simulink model "czujniki"  (R2013a)
settings: Solver=ode4  StartTime=0.0  StopTime=10  FixedStep=0.1  RelTol=1e-3
undefined symbols (not defined in the file or in its folder): serial
libraries: instrumentlib x2, dspindex x1
settings Model: Creator=Dzientak  LastModifiedBy=Dzientak

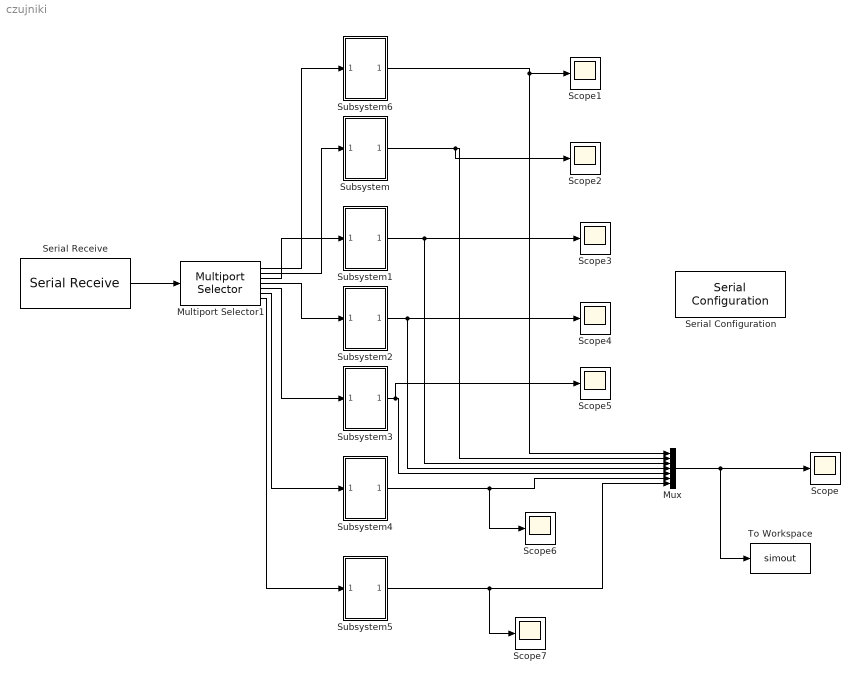
== system czujniki ==
  Multiport Selector1 : dspindex/Multiport Selector  rowsOrCols=Columns  idxCellArray={1,2,3,4,5,6,7 }  idxErrMode=Clip Index
  Mux : Mux  Inputs=7
  Scope{,1..7} (8 alike) : Scope
      Scope2 settings: SaveName=ScopeData2
      Scope3 settings: SaveName=ScopeData3
      Scope4 settings: SaveName=ScopeData4
      Scope5 settings: SaveName=ScopeData5
      Scope6 settings: SaveName=ScopeData6
      Scope7 settings: SaveName=ScopeData7
  Serial Configuration : instrumentlib/Serial Configuration  Priority=-200000  ComPortMenu=COM7  ComPort=COM7  ObjConstructor=serial('COM7');  BaudRate=9600  DataBits=8  Parity=none  StopBits=1  FlowControl=none  Timeout=10  ByteOrder=LittleEndian
  Serial Receive : instrumentlib/Serial Receive  ComPortMenu=COM7  ComPort=COM7  ObjConstructor=serial('COM7');  Terminator=<none>  DataSize="[8  7]"  DataType=uint8  EnableBlockingMode=on  ActionDataUnavailable=Output last received value  CustomValue=0  SampleTime=0.1
  Subsystem : Subsystem
  Subsystem1 : Subsystem
  Subsystem2 : Subsystem
  Subsystem3 : Subsystem
  Subsystem4 : Subsystem
  Subsystem5 : Subsystem
  Subsystem6 : Subsystem
  To Workspace : ToWorkspace  VariableName=simout  SampleTime=-1
  wires:
  Serial Receive/1 -> Multiport Selector1/1
  Multiport Selector1/1 -> Subsystem6/1(In1)
  Multiport Selector1/2 -> Subsystem/1(In1)
  Multiport Selector1/3 -> Subsystem1/1(In1)
  Multiport Selector1/4 -> Subsystem2/1(In1)
  Multiport Selector1/5 -> Subsystem3/1(In1)
  Multiport Selector1/6 -> Subsystem4/1(In1)
  Multiport Selector1/7 -> Subsystem5/1(In1)
  Subsystem6/1(Out1) -> Scope1/1, Mux/1
  Subsystem/1(Out1) -> Scope2/1, Mux/2
  Subsystem1/1(Out1) -> Scope3/1, Mux/3
  Subsystem2/1(Out1) -> Scope4/1, Mux/4
  Subsystem3/1(Out1) -> Scope5/1, Mux/5
  Subsystem4/1(Out1) -> Scope6/1, Mux/6
  Mux/1 -> To Workspace/1, Scope/1
  Subsystem5/1(Out1) -> Scope7/1, Mux/7

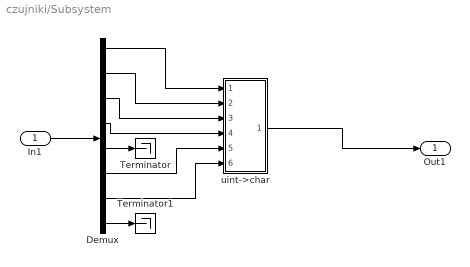
== system czujniki/Subsystem ==
  In1 : Inport
  Demux : Demux  Outputs=8
  Terminator : Terminator
  Terminator1 : Terminator
  uint->char : Subsystem
  Out1 : Outport
  wires:
  In1/1 -> Demux/1
  Demux/8 -> Terminator1/1
  Demux/5 -> Terminator/1
  Demux/7 -> uint->char/6(In6)
  Demux/6 -> uint->char/5(In5)
  Demux/4 -> uint->char/4(In4)
  Demux/3 -> uint->char/3(In3)
  Demux/2 -> uint->char/2(In2)
  Demux/1 -> uint->char/1(In1)
  uint->char/1(Out1) -> Out1/1

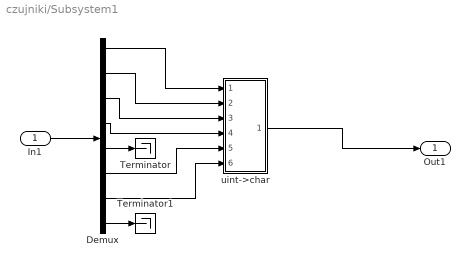
== system czujniki/Subsystem1 ==
  In1 : Inport
  Demux : Demux  Outputs=8
  Terminator : Terminator
  Terminator1 : Terminator
  uint->char : Subsystem
  Out1 : Outport
  wires:
  uint->char/1(Out1) -> Out1/1
  Demux/1 -> uint->char/1(In1)
  Demux/2 -> uint->char/2(In2)
  Demux/3 -> uint->char/3(In3)
  Demux/4 -> uint->char/4(In4)
  Demux/6 -> uint->char/5(In5)
  Demux/7 -> uint->char/6(In6)
  Demux/5 -> Terminator/1
  Demux/8 -> Terminator1/1
  In1/1 -> Demux/1

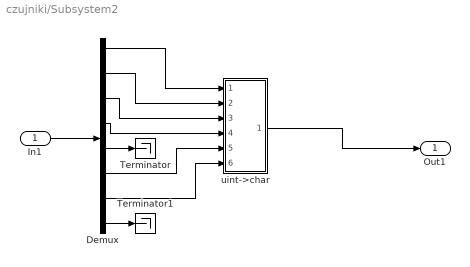
== system czujniki/Subsystem2 ==
  In1 : Inport
  Demux : Demux  Outputs=8
  Terminator : Terminator
  Terminator1 : Terminator
  uint->char : Subsystem
  Out1 : Outport
  wires:
  In1/1 -> Demux/1
  Demux/8 -> Terminator1/1
  Demux/5 -> Terminator/1
  Demux/7 -> uint->char/6(In6)
  Demux/6 -> uint->char/5(In5)
  Demux/4 -> uint->char/4(In4)
  Demux/3 -> uint->char/3(In3)
  Demux/2 -> uint->char/2(In2)
  Demux/1 -> uint->char/1(In1)
  uint->char/1(Out1) -> Out1/1

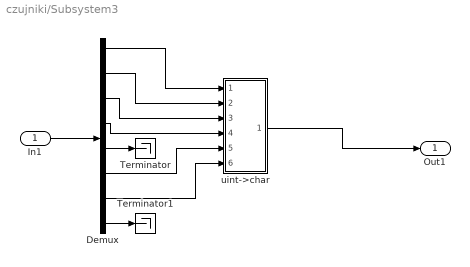
== system czujniki/Subsystem3 ==
  In1 : Inport
  Demux : Demux  Outputs=8
  Terminator : Terminator
  Terminator1 : Terminator
  uint->char : Subsystem
  Out1 : Outport
  wires:
  uint->char/1(Out1) -> Out1/1
  Demux/1 -> uint->char/1(In1)
  Demux/2 -> uint->char/2(In2)
  Demux/3 -> uint->char/3(In3)
  Demux/4 -> uint->char/4(In4)
  Demux/6 -> uint->char/5(In5)
  Demux/7 -> uint->char/6(In6)
  Demux/5 -> Terminator/1
  Demux/8 -> Terminator1/1
  In1/1 -> Demux/1

== system czujniki/Subsystem4 ==
  In1 : Inport
  Demux : Demux  Outputs=8
  Terminator : Terminator
  Terminator1 : Terminator
  uint->char : Subsystem
  Out1 : Outport
  wires:
  In1/1 -> Demux/1
  Demux/8 -> Terminator1/1
  Demux/5 -> Terminator/1
  Demux/7 -> uint->char/6(In6)
  Demux/6 -> uint->char/5(In5)
  Demux/4 -> uint->char/4(In4)
  Demux/3 -> uint->char/3(In3)
  Demux/2 -> uint->char/2(In2)
  Demux/1 -> uint->char/1(In1)
  uint->char/1(Out1) -> Out1/1

== system czujniki/Subsystem5 ==
  In1 : Inport
  Demux : Demux  Outputs=8
  Terminator : Terminator
  Terminator1 : Terminator
  uint->char : Subsystem
  Out1 : Outport
  wires:
  uint->char/1(Out1) -> Out1/1
  Demux/1 -> uint->char/1(In1)
  Demux/2 -> uint->char/2(In2)
  Demux/3 -> uint->char/3(In3)
  Demux/4 -> uint->char/4(In4)
  Demux/6 -> uint->char/5(In5)
  Demux/7 -> uint->char/6(In6)
  Demux/5 -> Terminator/1
  Demux/8 -> Terminator1/1
  In1/1 -> Demux/1

== system czujniki/Subsystem6 ==
  In1 : Inport
  Demux : Demux  Outputs=8
  Terminator : Terminator
  Terminator1 : Terminator
  uint->char : Subsystem
  Out1 : Outport
  wires:
  uint->char/1(Out1) -> Out1/1
  Demux/1 -> uint->char/1(In1)
  Demux/2 -> uint->char/2(In2)
  Demux/3 -> uint->char/3(In3)
  Demux/4 -> uint->char/4(In4)
  Demux/6 -> uint->char/5(In5)
  Demux/7 -> uint->char/6(In6)
  Demux/5 -> Terminator/1
  Demux/8 -> Terminator1/1
  In1/1 -> Demux/1

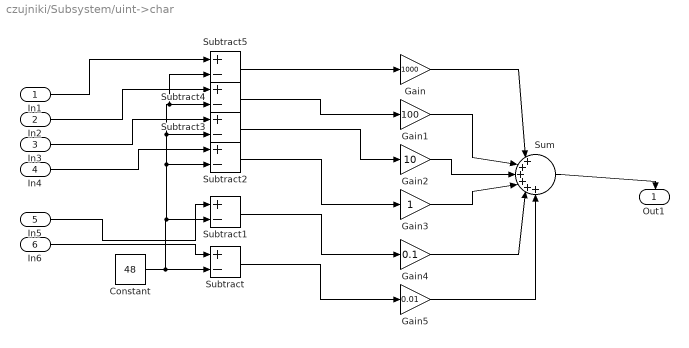
== system czujniki/Subsystem/uint->char ==
  In1 : Inport
  In2 : Inport  Port=2
  In3 : Inport  Port=3
  In4 : Inport  Port=4
  In5 : Inport  Port=5
  In6 : Inport  Port=6
  Constant : Constant  Value=48
  Gain : Gain  Gain=1000
  Gain1 : Gain  Gain=100
  Gain2 : Gain  Gain=10
  Gain3 : Gain
  Gain4 : Gain  Gain=0.1
  Gain5 : Gain  Gain=0.01
  Subtract{,1..5} (6 alike) : Sum  Inputs=+-
  Sum : Sum  Inputs=|++++++
  Out1 : Outport
  wires:
  In3/1 -> Subtract3/1
  Constant/1 -> Subtract5/2, Subtract4/2, Subtract3/2, Subtract2/2, Subtract1/2, Subtract/2
  In6/1 -> Subtract/1
  In2/1 -> Subtract4/1
  In1/1 -> Subtract5/1
  In4/1 -> Subtract2/1
  In5/1 -> Subtract1/1
  Subtract/1 -> Gain5/1
  Subtract1/1 -> Gain4/1
  Subtract2/1 -> Gain3/1
  Subtract3/1 -> Gain2/1
  Subtract4/1 -> Gain1/1
  Subtract5/1 -> Gain/1
  Gain/1 -> Sum/1
  Gain1/1 -> Sum/2
  Gain2/1 -> Sum/3
  Gain3/1 -> Sum/4
  Gain4/1 -> Sum/5
  Gain5/1 -> Sum/6
  Sum/1 -> Out1/1

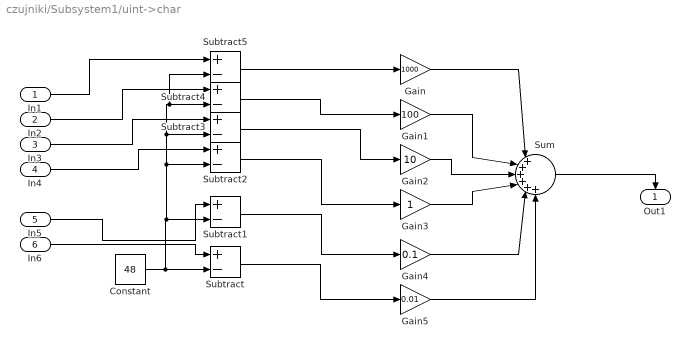
== system czujniki/Subsystem1/uint->char ==
  In1 : Inport
  In2 : Inport  Port=2
  In3 : Inport  Port=3
  In4 : Inport  Port=4
  In5 : Inport  Port=5
  In6 : Inport  Port=6
  Constant : Constant  Value=48
  Gain : Gain  Gain=1000
  Gain1 : Gain  Gain=100
  Gain2 : Gain  Gain=10
  Gain3 : Gain
  Gain4 : Gain  Gain=0.1
  Gain5 : Gain  Gain=0.01
  Subtract{,1..5} (6 alike) : Sum  Inputs=+-
  Sum : Sum  Inputs=|++++++
  Out1 : Outport
  wires:
  Sum/1 -> Out1/1
  Gain5/1 -> Sum/6
  Gain4/1 -> Sum/5
  Gain3/1 -> Sum/4
  Gain2/1 -> Sum/3
  Gain1/1 -> Sum/2
  Gain/1 -> Sum/1
  Subtract5/1 -> Gain/1
  Subtract4/1 -> Gain1/1
  Subtract3/1 -> Gain2/1
  Subtract2/1 -> Gain3/1
  Subtract1/1 -> Gain4/1
  Subtract/1 -> Gain5/1
  In5/1 -> Subtract1/1
  In4/1 -> Subtract2/1
  In1/1 -> Subtract5/1
  In2/1 -> Subtract4/1
  In6/1 -> Subtract/1
  Constant/1 -> Subtract/2, Subtract1/2, Subtract2/2, Subtract3/2, Subtract4/2, Subtract5/2
  In3/1 -> Subtract3/1

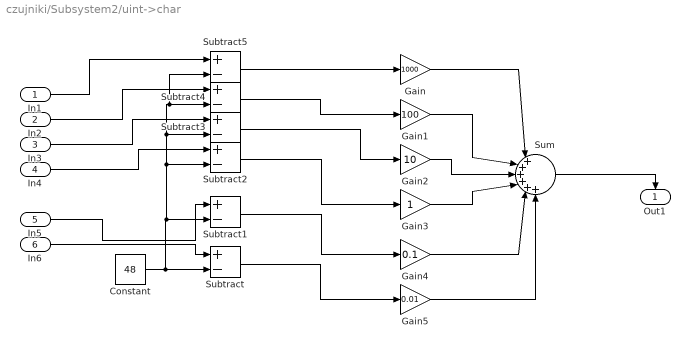
== system czujniki/Subsystem2/uint->char ==
  In1 : Inport
  In2 : Inport  Port=2
  In3 : Inport  Port=3
  In4 : Inport  Port=4
  In5 : Inport  Port=5
  In6 : Inport  Port=6
  Constant : Constant  Value=48
  Gain : Gain  Gain=1000
  Gain1 : Gain  Gain=100
  Gain2 : Gain  Gain=10
  Gain3 : Gain
  Gain4 : Gain  Gain=0.1
  Gain5 : Gain  Gain=0.01
  Subtract{,1..5} (6 alike) : Sum  Inputs=+-
  Sum : Sum  Inputs=|++++++
  Out1 : Outport
  wires:
  In3/1 -> Subtract3/1
  Constant/1 -> Subtract5/2, Subtract4/2, Subtract3/2, Subtract2/2, Subtract1/2, Subtract/2
  In6/1 -> Subtract/1
  In2/1 -> Subtract4/1
  In1/1 -> Subtract5/1
  In4/1 -> Subtract2/1
  In5/1 -> Subtract1/1
  Subtract/1 -> Gain5/1
  Subtract1/1 -> Gain4/1
  Subtract2/1 -> Gain3/1
  Subtract3/1 -> Gain2/1
  Subtract4/1 -> Gain1/1
  Subtract5/1 -> Gain/1
  Gain/1 -> Sum/1
  Gain1/1 -> Sum/2
  Gain2/1 -> Sum/3
  Gain3/1 -> Sum/4
  Gain4/1 -> Sum/5
  Gain5/1 -> Sum/6
  Sum/1 -> Out1/1

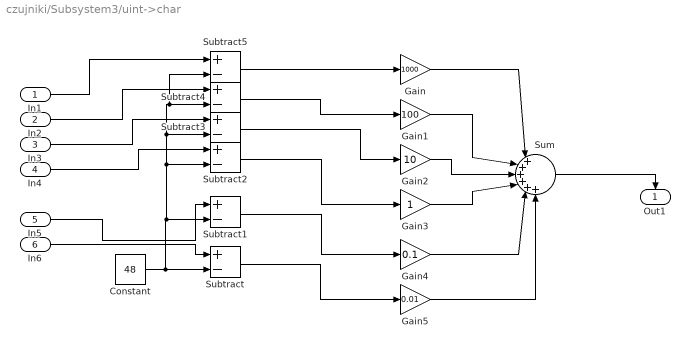
== system czujniki/Subsystem3/uint->char ==
  In1 : Inport
  In2 : Inport  Port=2
  In3 : Inport  Port=3
  In4 : Inport  Port=4
  In5 : Inport  Port=5
  In6 : Inport  Port=6
  Constant : Constant  Value=48
  Gain : Gain  Gain=1000
  Gain1 : Gain  Gain=100
  Gain2 : Gain  Gain=10
  Gain3 : Gain
  Gain4 : Gain  Gain=0.1
  Gain5 : Gain  Gain=0.01
  Subtract{,1..5} (6 alike) : Sum  Inputs=+-
  Sum : Sum  Inputs=|++++++
  Out1 : Outport
  wires:
  Sum/1 -> Out1/1
  Gain5/1 -> Sum/6
  Gain4/1 -> Sum/5
  Gain3/1 -> Sum/4
  Gain2/1 -> Sum/3
  Gain1/1 -> Sum/2
  Gain/1 -> Sum/1
  Subtract5/1 -> Gain/1
  Subtract4/1 -> Gain1/1
  Subtract3/1 -> Gain2/1
  Subtract2/1 -> Gain3/1
  Subtract1/1 -> Gain4/1
  Subtract/1 -> Gain5/1
  In5/1 -> Subtract1/1
  In4/1 -> Subtract2/1
  In1/1 -> Subtract5/1
  In2/1 -> Subtract4/1
  In6/1 -> Subtract/1
  Constant/1 -> Subtract/2, Subtract1/2, Subtract2/2, Subtract3/2, Subtract4/2, Subtract5/2
  In3/1 -> Subtract3/1

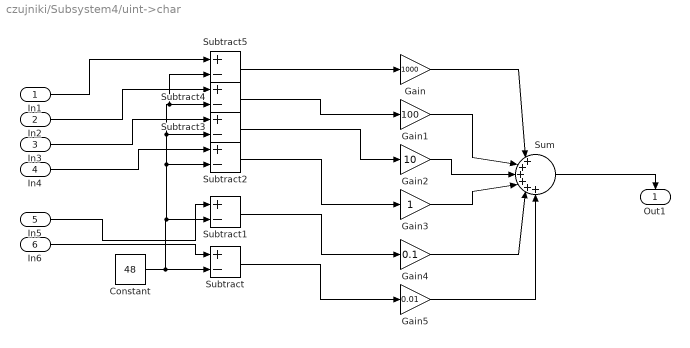
== system czujniki/Subsystem4/uint->char ==
  In1 : Inport
  In2 : Inport  Port=2
  In3 : Inport  Port=3
  In4 : Inport  Port=4
  In5 : Inport  Port=5
  In6 : Inport  Port=6
  Constant : Constant  Value=48
  Gain : Gain  Gain=1000
  Gain1 : Gain  Gain=100
  Gain2 : Gain  Gain=10
  Gain3 : Gain
  Gain4 : Gain  Gain=0.1
  Gain5 : Gain  Gain=0.01
  Subtract{,1..5} (6 alike) : Sum  Inputs=+-
  Sum : Sum  Inputs=|++++++
  Out1 : Outport
  wires:
  In3/1 -> Subtract3/1
  Constant/1 -> Subtract5/2, Subtract4/2, Subtract3/2, Subtract2/2, Subtract1/2, Subtract/2
  In6/1 -> Subtract/1
  In2/1 -> Subtract4/1
  In1/1 -> Subtract5/1
  In4/1 -> Subtract2/1
  In5/1 -> Subtract1/1
  Subtract/1 -> Gain5/1
  Subtract1/1 -> Gain4/1
  Subtract2/1 -> Gain3/1
  Subtract3/1 -> Gain2/1
  Subtract4/1 -> Gain1/1
  Subtract5/1 -> Gain/1
  Gain/1 -> Sum/1
  Gain1/1 -> Sum/2
  Gain2/1 -> Sum/3
  Gain3/1 -> Sum/4
  Gain4/1 -> Sum/5
  Gain5/1 -> Sum/6
  Sum/1 -> Out1/1

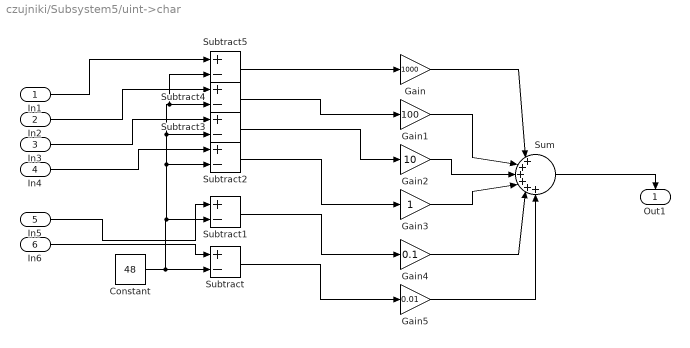
== system czujniki/Subsystem5/uint->char ==
  In1 : Inport
  In2 : Inport  Port=2
  In3 : Inport  Port=3
  In4 : Inport  Port=4
  In5 : Inport  Port=5
  In6 : Inport  Port=6
  Constant : Constant  Value=48
  Gain : Gain  Gain=1000
  Gain1 : Gain  Gain=100
  Gain2 : Gain  Gain=10
  Gain3 : Gain
  Gain4 : Gain  Gain=0.1
  Gain5 : Gain  Gain=0.01
  Subtract{,1..5} (6 alike) : Sum  Inputs=+-
  Sum : Sum  Inputs=|++++++
  Out1 : Outport
  wires:
  Sum/1 -> Out1/1
  Gain5/1 -> Sum/6
  Gain4/1 -> Sum/5
  Gain3/1 -> Sum/4
  Gain2/1 -> Sum/3
  Gain1/1 -> Sum/2
  Gain/1 -> Sum/1
  Subtract5/1 -> Gain/1
  Subtract4/1 -> Gain1/1
  Subtract3/1 -> Gain2/1
  Subtract2/1 -> Gain3/1
  Subtract1/1 -> Gain4/1
  Subtract/1 -> Gain5/1
  In5/1 -> Subtract1/1
  In4/1 -> Subtract2/1
  In1/1 -> Subtract5/1
  In2/1 -> Subtract4/1
  In6/1 -> Subtract/1
  Constant/1 -> Subtract/2, Subtract1/2, Subtract2/2, Subtract3/2, Subtract4/2, Subtract5/2
  In3/1 -> Subtract3/1

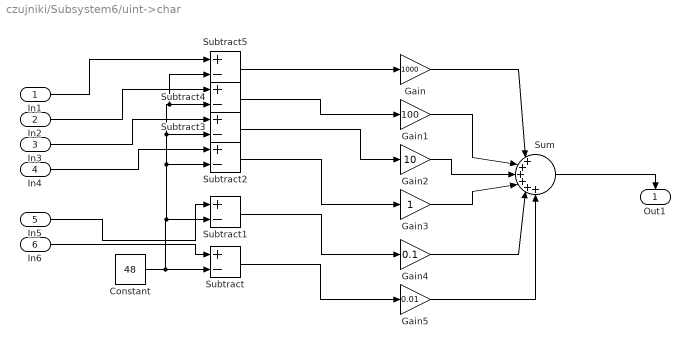
== system czujniki/Subsystem6/uint->char ==
  In1 : Inport
  In2 : Inport  Port=2
  In3 : Inport  Port=3
  In4 : Inport  Port=4
  In5 : Inport  Port=5
  In6 : Inport  Port=6
  Constant : Constant  Value=48
  Gain : Gain  Gain=1000
  Gain1 : Gain  Gain=100
  Gain2 : Gain  Gain=10
  Gain3 : Gain
  Gain4 : Gain  Gain=0.1
  Gain5 : Gain  Gain=0.01
  Subtract{,1..5} (6 alike) : Sum  Inputs=+-
  Sum : Sum  Inputs=|++++++
  Out1 : Outport
  wires:
  Sum/1 -> Out1/1
  Gain5/1 -> Sum/6
  Gain4/1 -> Sum/5
  Gain3/1 -> Sum/4
  Gain2/1 -> Sum/3
  Gain1/1 -> Sum/2
  Gain/1 -> Sum/1
  Subtract5/1 -> Gain/1
  Subtract4/1 -> Gain1/1
  Subtract3/1 -> Gain2/1
  Subtract2/1 -> Gain3/1
  Subtract1/1 -> Gain4/1
  Subtract/1 -> Gain5/1
  In5/1 -> Subtract1/1
  In4/1 -> Subtract2/1
  In1/1 -> Subtract5/1
  In2/1 -> Subtract4/1
  In6/1 -> Subtract/1
  Constant/1 -> Subtract/2, Subtract1/2, Subtract2/2, Subtract3/2, Subtract4/2, Subtract5/2
  In3/1 -> Subtract3/1
